simulink model "Vehicle1D_harness_model"  (R2022a)
settings: Solver=daessc  StartTime=0.0  StopTime=t_end  RelTol=1e-3  AbsTol=1e-3
PreLoadFcn:
  | Vehicle1D_harness_setup
undefined symbols (not defined in the file or in its folder): gearTrain
libraries: fl_lib x5, nesl_utility x2
settings Model: Creator=isaacito  LastModifiedBy=isaacito
settings SolverCC: AutoScaleAbsTol=off  AlgebraicLoopSolver=TrustRegion
settings DebuggingCC: UnconnectedInputMsg=warning  UnconnectedOutputMsg=warning  UnconnectedLineMsg=warning  SFMachineParentedDataDiag=warning
settings RTWCC: DLArmComputeVersion=19.05
settings SimscapeCC: SimscapeLogType=all  SimscapeLogSimulationStatistics=on  SimscapeLogLimitData=off

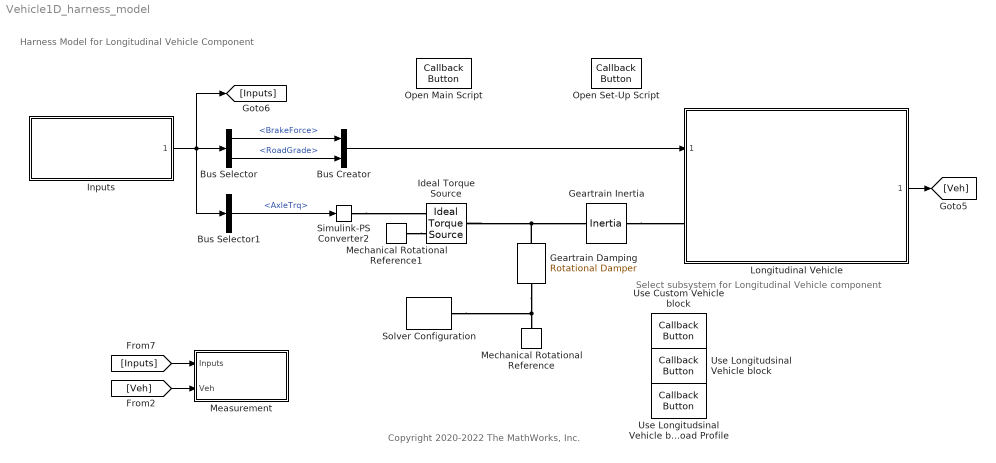
== system Vehicle1D_harness_model ==
  note: Select subsystem for Longitudinal Vehicle component
  note: Harness Model for Longitudinal Vehicle Component
  note: Copyright 2020-2022 The MathWorks, Inc.
  Bus Creator : BusCreator  Inputs=2
  Bus Selector : BusSelector  OutputSignals=BrakeForce,RoadGrade
  Bus Selector1 : BusSelector  OutputSignals=AxleTrq
  Geartrain Damping : fl_lib/Mechanical/Rotational Elements/Rotational Damper  D=gearTrain.friction_Nm_per_rpm m*N/rpm  w_specify=off  w_priority=None  w=0 rad/s  w_nominal_specify=off  w_nominal_unit=rad/s  w_nominal_value=1  t_specify=off  t_priority=None  t=0 N*m  t_nominal_specify=off  t_nominal_unit=N*m  t_nominal_value=1
      settings: SourceProductBaseCode=PW,SS,VE
      settings: AttributesFormatString=|
      | %<D>
      | %<D_unit>
  Geartrain Inertia : fl_lib/Mechanical/Rotational Elements/Inertia  inertia=gearTrain.inertia_kg_m2 kg*m^2  num_ports=foundation.enum.numPorts2.two  w_specify=on  w_priority=None  w=0 rpm  w_nominal_specify=off  w_nominal_unit=rad/s  w_nominal_value=1  t_specify=off  t_priority=None  t=0 N*m  t_nominal_specify=off  t_nominal_unit=N*m  t_nominal_value=1
      settings: SourceProductBaseCode=PW,SS,VE  InternalSimscapePortConfiguration="{\"Bottom\":[],\"Left\":[{\"id\":\"I\",\"label\":\"\",\"type\":\"foundation.mechanical.rotational.rotational\"}],\"Right\":[{\"id\":\"J\",\"label\":\"\",\"type\":\"foundation.mechanical.rotational.rotational\"}],\"Top\":[]}"
      settings: AttributesFormatString=|
      | %<inertia>
      | %<inertia_unit>
  Ideal Torque Source : fl_lib/Mechanical/Mechanical Sources/Ideal Torque Source
      settings: SourceProductBaseCode=PW,SS,VE
  Inputs : Subsystem  ReferencedSubsystem=Vehicle1D_input_refsub
  Longitudinal Vehicle : Subsystem  ReferencedSubsystem=Vehicle1D_refsub_Driveline
  Measurement : Subsystem
  Mechanical Rotational Reference : fl_lib/Mechanical/Rotational Elements/Mechanical Rotational Reference
      settings: SourceProductBaseCode=PW,SS,VE
  Mechanical Rotational Reference1 : fl_lib/Mechanical/Rotational Elements/Mechanical Rotational Reference
      settings: SourceProductBaseCode=PW,SS,VE
  Open Main Script : CallbackButton  ButtonText=Open
      settings: ClickFcn=edit Vehicle1D_main_script
  Open Set-Up Script : CallbackButton  ButtonText=Open
      settings: ClickFcn=edit Vehicle1D_harness_setup
  Simulink-PS Converter2 : nesl_utility/Simulink-PS Converter  PhysicalDomain=network_engine_domain  SubClassName=ps_input  LeftPortType=input  RightPortType=output  PseudoPeriodic=off  Frequencies=[]  NoiseDistribution=none  NoiseParameters=[]  Unit=N*m  AffineConversion=off  FilteringAndDerivatives=filter  SimscapeFilterOrder=1  InputFilterTimeConstant=0.001  UdotUserProvided=0
      settings: SourceProductBaseCode=SS,PW,VE
  Solver Configuration : nesl_utility/Solver Configuration  PhysicalDomain=network_engine_domain  SubClassName=solver  LeftPortType=input  RightPortType=generic  Tones=[]  Harmonics=[]  SimulateNoise=off  Profile=off  UseLocalSampling=off  EnableSwitchedLinearOptims=on  FrequencyDomain=off  UseCCode=off  RelTol=0.001  AbsTol=1e-06  MinStep=1e-09  ToWorkspace=off  RevertToSquareIcSolve=off  NumHomotopyIterations=100  PhasorMode=off  PhasorModeNumHarmonics=1  IndexReductionMethod=DerivativeReplacement  DoDC=off  ResidualTolerance=1e-09  UseLocalSolver=off  LocalSolverChoice=NE_BACKWARD_EULER_ADVANCER  LocalSolverSampleTime=0.001  DoFixedCost=off  MaxNonlinIter=3  MaxModeIter=2  ComputeImpulses=off  ImpulseIterations=2  LinearAlgebra=auto  LinearAlgebraNumThread=0  EquationFormulation=NE_TIME_EF  DelaysMemoryBudget=1024  AutomaticFiltering=on  FilteringTimeConstant=0.001  PartitionStorageMethod=AS_NEEDED  PartitionMemoryBudget=1024  PartitionMethod=ROBUST
      settings: AttributesFormatString=Local solver %<UseLocalSolver>  SourceProductBaseCode=SS,PW,VE
  Use Custom Vehicle block : CallbackButton  ButtonText=Select
      settings: ClickFcn=|
      | blkpath = "/Longitudinal Vehicle";
      | set_param( gcs + blkpath, ...
      |   ReferencedSubsystem = ...
      |   "Vehicle1D_refsub_Custom");
  Use Longitudsinal Vehicle block : CallbackButton  ButtonText=Select
      settings: ClickFcn=|
      | blkpath = "/Longitudinal Vehicle";
      | set_param( gcs + blkpath, ...
      |   ReferencedSubsystem = ...
      |   "Vehicle1D_refsub_Driveline");
  Use Longitudsinal Vehicle block with Road Profile : CallbackButton  ButtonText=Select
      settings: ClickFcn=|
      | blkpath = "/Longitudinal Vehicle";
      | set_param( gcs + blkpath, ...
      |   ReferencedSubsystem = ...
      |   "Vehicle1D_refsub_Driveline_withRoadProfile");
  wires:
  Longitudinal Vehicle/1 -> [Veh]
  [Veh] -> Measurement/2(Veh)
  [Inputs] -> Measurement/1(Inputs)
  Inputs/1 -> Bus Selector1/1, [Inputs], Bus Selector/1
  Bus Creator/1 -> Longitudinal Vehicle/1
  Bus Selector1/1 -> Simulink-PS Converter2/1  "<AxleTrq>"
  Bus Selector/1 -> Bus Creator/1  "<BrakeForce>"
  Bus Selector/2 -> Bus Creator/2  "<RoadGrade>"
  connections:
  Geartrain Damping/RConn1 -- Solver Configuration/RConn1 -- Mechanical Rotational Reference/LConn1
  Mechanical Rotational Reference1/LConn1 -- Ideal Torque Source/RConn2
  Geartrain Inertia/LConn1 -- Longitudinal Vehicle/LConn1
  Ideal Torque Source/LConn1 -- Geartrain Damping/LConn1 -- Geartrain Inertia/RConn1
  Simulink-PS Converter2/RConn1 -- Ideal Torque Source/RConn1

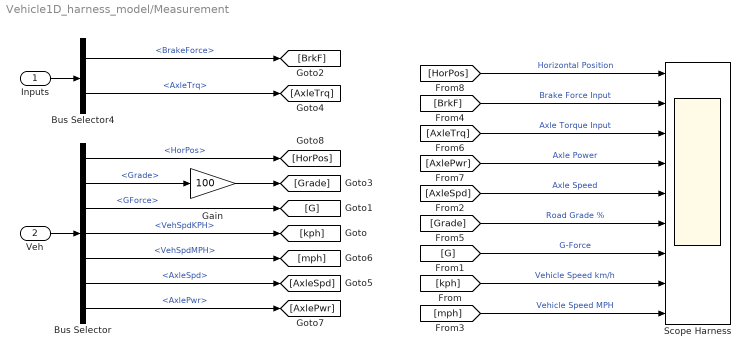
== system Vehicle1D_harness_model/Measurement ==
  Inputs : Inport
  Veh : Inport  Port=2
  Bus Selector : BusSelector  OutputSignals=HorPos,Grade,GForce,VehSpdKPH,VehSpdMPH,AxleSpd,AxlePwr
  Bus Selector4 : BusSelector  OutputSignals=BrakeForce,AxleTrq
  Gain : Gain  Gain=100
  Scope Harness : Scope  NumInputPorts=9
  wires:
  Inputs/1 -> Bus Selector4/1
  Veh/1 -> Bus Selector/1
  Bus Selector4/1 -> [BrkF]  "<BrakeForce>"
  Bus Selector4/2 -> [AxleTrq]  "<AxleTrq>"
  Bus Selector/2 -> Gain/1  "<Grade>"
  Bus Selector/3 -> [G]  "<GForce>"
  Bus Selector/4 -> [kph]  "<VehSpdKPH>"
  Bus Selector/5 -> [mph]  "<VehSpdMPH>"
  Bus Selector/6 -> [AxleSpd]  "<AxleSpd>"
  Bus Selector/7 -> [AxlePwr]  "<AxlePwr>"
  Gain/1 -> [Grade]
  Bus Selector/1 -> [HorPos]  "<HorPos>"
  [HorPos] -> Scope Harness/1  "Horizontal Position"
  [BrkF] -> Scope Harness/2  "Brake Force Input"
  [AxleTrq] -> Scope Harness/3  "Axle Torque Input"
  [AxlePwr] -> Scope Harness/4  "Axle Power"
  [AxleSpd] -> Scope Harness/5  "Axle Speed"
  [Grade] -> Scope Harness/6  "Road Grade %"
  [G] -> Scope Harness/7  "G-Force"
  [kph] -> Scope Harness/8  "Vehicle Speed km/h"
  [mph] -> Scope Harness/9  "Vehicle Speed MPH"
